simulink subsystem "ServicingSatGNC"  (R2023a)
settings: Solver=VariableStepAuto  StartTime=0.0  StopTime=10.0  RelTol=1e-3
undefined symbols (not defined in the file or in its folder): jointControlData
settings Model: Creator=Andy  LastModifiedBy=Andy
settings OptimizationCC: ReuseModelBlockBuffer=off
settings ModelReferenceCC: EnableRefExpFcnMdlSchedulingChecks=on

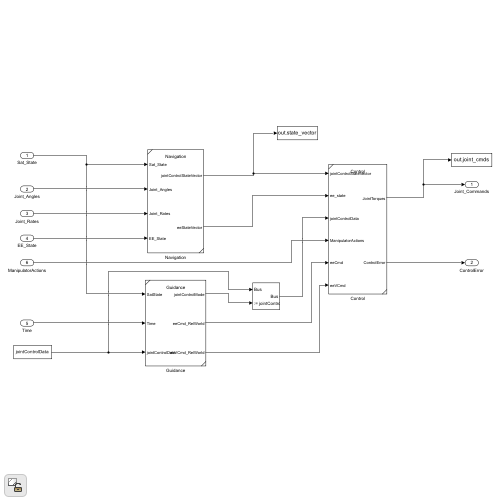
[thumbnail: Simulink's stored preview of the top-level diagram]
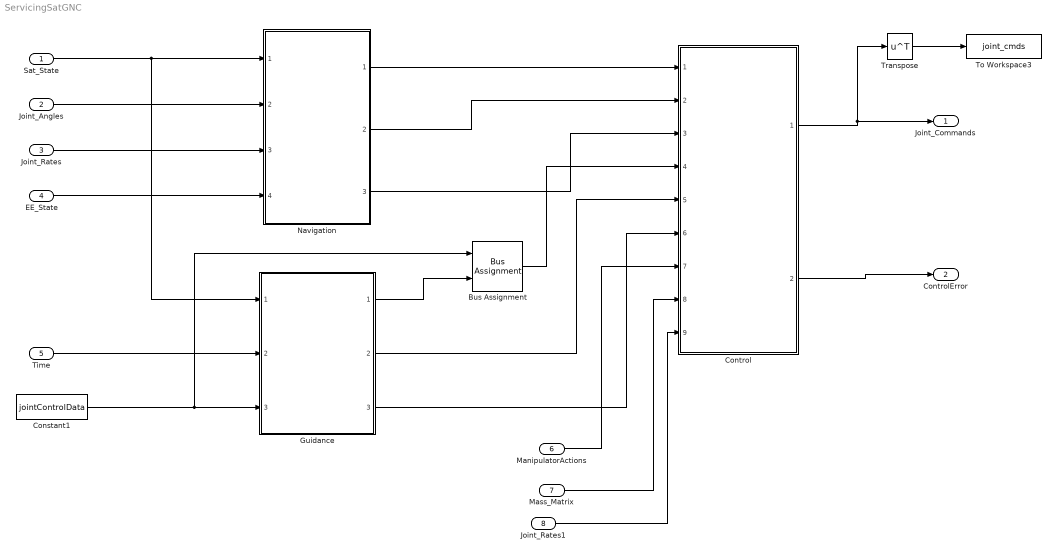
== system ServicingSatGNC ==
  Sat_State : Inport
  Joint_Angles : Inport  Port=2
  Joint_Rates : Inport  Port=3
  EE_State : Inport  Port=4
  Time : Inport  Port=5
  ManipulatorActions : Inport  Port=6
  Mass_Matrix : Inport  Port=7
  Joint_Rates1 : Inport  Port=8
  Bus Assignment : BusAssignment  AssignedSignals=jointControlMode
  Constant1 : Constant  Value=jointControlData  OutDataTypeStr=Bus:jointControlDataBus
  Control : Subsystem  ReferencedSubsystem=Control
  Guidance : Subsystem  ReferencedSubsystem=Guidance
  Navigation : Subsystem  ReferencedSubsystem=Navigation
  To Workspace3 : ToWorkspace  VariableName=joint_cmds  SaveFormat=Timeseries  SampleTime=-1
  Transpose : Math  Operator=transpose
  Joint_Commands : Outport
  ControlError : Outport  Port=2
  wires:
  Sat_State/1 -> Navigation/1, Guidance/1
  EE_State/1 -> Navigation/4
  Navigation/3 -> Control/3
  Constant1/1 -> Guidance/3, Bus Assignment/1
  Bus Assignment/1 -> Control/4
  Time/1 -> Guidance/2
  Control/1 -> Joint_Commands/1, Transpose/1
  Guidance/1 -> Bus Assignment/2
  ManipulatorActions/1 -> Control/7
  Control/2 -> ControlError/1
  Guidance/2 -> Control/5
  Guidance/3 -> Control/6
  Joint_Angles/1 -> Navigation/2
  Joint_Rates/1 -> Navigation/3
  Mass_Matrix/1 -> Control/8
  Navigation/1 -> Control/1
  Navigation/2 -> Control/2
  Transpose/1 -> To Workspace3/1
  Joint_Rates1/1 -> Control/9
